simulink model "robotarm_generalization_error"  (R2018b)
settings: Solver=FixedStepAuto  StartTime=0.0  StopTime=10  FixedStep=options.dt  RelTol=1e-3  AbsTol=1e-6
PreLoadFcn:
  | const_ref=-0.1;
  | options.dt=0.02;
libraries: neural x528, simulink x1
(part 6 of 20)

== system robotarm_generalization_error/pre_0/Layer 3/Delays 1 ==
  "p{3}" : Inport  PortDimensions=30
      mask Display: e = 0.06;c1 = [120 230 180]/255;c2 = ([120 230 180]+0)/(256+128);c3 = ([120 230 180]+128)/(256+128);patch([0 1 1 0],[0 0 1 1],c1);patch([0 1 1 1-e 1-e 0+e],[0 0 1 1-e 0+e 0+e],c2);patch([0 0 1 1-e 0+e 0+e],[0 1 1 1-e 1-e 0+e],c3);plot([0 1 1 0 0],[0 0 1 1 0]);
  mux : Mux  Inputs=1
      mask Display: e = 0.06;c1 = [120 150 230]/255;c2 = ([120 150 230]+0)/383;c3 = ([120 150 230]+128)/383;patch([0 1 1 0],[0 0 1 1],c1);patch([0 1 1 1-e 1-e 0+e],[0 0 1 1-e 0+e 0+e],c2);patch([0 0 1 1-e 0+e 0+e],[0 1 1 1-e 1-e 0+e],c3);plot([0 1 1 0 0],[0 0 1 1 0]);disp('Mux')
  "pd{3,2}" : Outport
      mask Display: e = 0.06;c1 = [120 230 180]/255;c2 = ([120 230 180]+0)/(256+128);c3 = ([120 230 180]+128)/(256+128);patch([0 1 1 0],[0 0 1 1],c1);patch([0 1 1 1-e 1-e 0+e],[0 0 1 1-e 0+e 0+e],c2);patch([0 0 1 1-e 0+e 0+e],[0 1 1 1-e 1-e 0+e],c3);plot([0 1 1 0 0],[0 0 1 1 0]);
  wires:
  "p{3}"/1 -> mux/1
  mux/1 -> "pd{3,2}"/1

== system robotarm_generalization_error/pre_0/Layer 3/LW{3,2} ==
  "ad{3,2}" : Inport  PortDimensions=30
      mask Display: e = 0.06;c1 = [120 230 180]/255;c2 = ([120 230 180]+0)/(256+128);c3 = ([120 230 180]+128)/(256+128);patch([0 1 1 0],[0 0 1 1],c1);patch([0 1 1 1-e 1-e 0+e],[0 0 1 1-e 0+e 0+e],c2);patch([0 0 1 1-e 0+e 0+e],[0 1 1 1-e 1-e 0+e],c3);plot([0 1 1 0 0],[0 0 1 1 0]);
  "IW{3,2}(1,:)'" : Constant  Value=[0.1482283738558132502038944267042097635567188262939453125;-0.292502547224109787915580227490863762795925140380859375;-0.50468612294941428420003148858086206018924713134765625;-0.04670559747562709473900355305886478163301944732666015625;-0.041057504134613953539201247622258961200714111328125;-0.047944240213243671799858702797791920602321624755859375;-0.058496921474289344244912314252360374666750431060791015625;0.6148107235436384154780853350530378520488739013671875;0.426521583356435696199326912392280064523220062255859375;-0.07561076580819027503910234599970863200724124908447265625;-0.11443132652669028848091414829468703828752040863037109375;0.0323020095753548119876796818061848171055316925048828125;-0.09697924204691467375827329533422016538679599761962890625;-0.0005858338048831922273418371105435653589665889739990234375;0.401630644371972878037269083506544120609760284423828125;-0.01411896694504084781573993723213789053261280059814453125;0.128668160799946307282226598545094020664691925048828125;0.315585885323380666012127448993851430714130401611328125;0.03498763759822243191166535325464792549610137939453125;0.263939485164793652405279544836957938969135284423828125;-0.04660773546215137008719153755009756423532962799072265625;0.098416358531250913710408667611773125827312469482421875;-0.05026154890612459513743459638135391287505626678466796875;0.5797294681370976920931070708320476114749908447265625;-0.1274272878263316977065500168464495800435543060302734375;0.29329703665639728082936699138372205197811126708984375;-0.20780235218750531256404201485565863549709320068359375;0.1349574147376667310194164883796474896371364593505859375;0.158832086422066420805521147485706023871898651123046875;-0.38523169250914823802389719276106916368007659912109375]
      mask Display: e = 0.06;c1 = [120 150 230]/255;c2 = ([120 150 230]+0)/383;c3 = ([120 150 230]+128)/383;patch([0 1 1 0],[0 0 1 1],c1);patch([0 1 1 1-e 1-e 0+e],[0 0 1 1-e 0+e 0+e],c2);patch([0 0 1 1-e 0+e 0+e],[0 1 1 1-e 1-e 0+e],c3);plot([0 1 1 0 0],[0 0 1 1 0]);disp('weights');
  Mux : Mux  Inputs=1
      mask Display: e = 0.06;c1 = [120 150 230]/255;c2 = ([120 150 230]+0)/383;c3 = ([120 150 230]+128)/383;patch([0 1 1 0],[0 0 1 1],c1);patch([0 1 1 1-e 1-e 0+e],[0 0 1 1-e 0+e 0+e],c2);patch([0 0 1 1-e 0+e 0+e],[0 1 1 1-e 1-e 0+e],c3);plot([0 1 1 0 0],[0 0 1 1 0]);disp('Mux');
  dotprod1 : neural/Weight Functions/dotprod
  "lz{3,2}" : Outport
      mask Display: e = 0.06;c1 = [120 230 180]/255;c2 = ([120 230 180]+0)/(256+128);c3 = ([120 230 180]+128)/(256+128);patch([0 1 1 0],[0 0 1 1],c1);patch([0 1 1 1-e 1-e 0+e],[0 0 1 1-e 0+e 0+e],c2);patch([0 0 1 1-e 0+e 0+e],[0 1 1 1-e 1-e 0+e],c3);plot([0 1 1 0 0],[0 0 1 1 0]);
  wires:
  "IW{3,2}(1,:)'"/1 -> dotprod1/1
  "ad{3,2}"/1 -> dotprod1/2
  dotprod1/1 -> Mux/1
  Mux/1 -> "lz{3,2}"/1

== system robotarm_generalization_error/pre_0.00001/Layer 1/Delays 1 ==
  "p{1}" : Inport  PortDimensions=10
      mask Display: e = 0.06;c1 = [120 230 180]/255;c2 = ([120 230 180]+0)/(256+128);c3 = ([120 230 180]+128)/(256+128);patch([0 1 1 0],[0 0 1 1],c1);patch([0 1 1 1-e 1-e 0+e],[0 0 1 1-e 0+e 0+e],c2);patch([0 0 1 1-e 0+e 0+e],[0 1 1 1-e 1-e 0+e],c3);plot([0 1 1 0 0],[0 0 1 1 0]);
  mux : Mux  Inputs=1
      mask Display: e = 0.06;c1 = [120 150 230]/255;c2 = ([120 150 230]+0)/383;c3 = ([120 150 230]+128)/383;patch([0 1 1 0],[0 0 1 1],c1);patch([0 1 1 1-e 1-e 0+e],[0 0 1 1-e 0+e 0+e],c2);patch([0 0 1 1-e 0+e 0+e],[0 1 1 1-e 1-e 0+e],c3);plot([0 1 1 0 0],[0 0 1 1 0]);disp('Mux')
  "pd{1,1}" : Outport
      mask Display: e = 0.06;c1 = [120 230 180]/255;c2 = ([120 230 180]+0)/(256+128);c3 = ([120 230 180]+128)/(256+128);patch([0 1 1 0],[0 0 1 1],c1);patch([0 1 1 1-e 1-e 0+e],[0 0 1 1-e 0+e 0+e],c2);patch([0 0 1 1-e 0+e 0+e],[0 1 1 1-e 1-e 0+e],c3);plot([0 1 1 0 0],[0 0 1 1 0]);
  wires:
  "p{1}"/1 -> mux/1
  mux/1 -> "pd{1,1}"/1

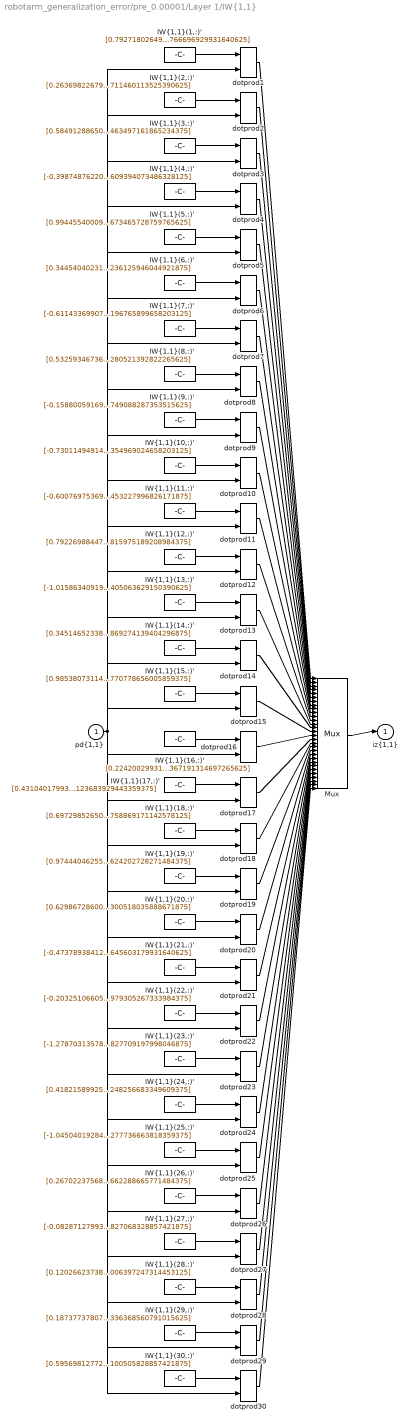
== system robotarm_generalization_error/pre_0.00001/Layer 1/IW{1,1} ==
  "pd{1,1}" : Inport  PortDimensions=10
      mask Display: e = 0.06;c1 = [120 230 180]/255;c2 = ([120 230 180]+0)/(256+128);c3 = ([120 230 180]+128)/(256+128);patch([0 1 1 0],[0 0 1 1],c1);patch([0 1 1 1-e 1-e 0+e],[0 0 1 1-e 0+e 0+e],c2);patch([0 0 1 1-e 0+e 0+e],[0 1 1 1-e 1-e 0+e],c3);plot([0 1 1 0 0],[0 0 1 1 0]);
  "IW{1,1}(1,:)'" : Constant  Value=[0.792718026499978467569462736719287931919097900390625;-0.70093126819101170266179678947082720696926116943359375;0.05608783841132684855335099882722715847194194793701171875;0.650494068864035934751655076979659497737884521484375;0.339334487435024423351848099628114141523838043212890625;0.0859367098609566948397286978433839976787567138671875;-0.00303800444739509879765737565548988641239702701568603515625;0.403054897202263173738856494310311973094940185546875;-0.9987802927080036141660457360558211803436279296875;0.88997533042789600532529448173590935766696929931640625]
      mask Display: e = 0.06;c1 = [120 150 230]/255;c2 = ([120 150 230]+0)/383;c3 = ([120 150 230]+128)/383;patch([0 1 1 0],[0 0 1 1],c1);patch([0 1 1 1-e 1-e 0+e],[0 0 1 1-e 0+e 0+e],c2);patch([0 0 1 1-e 0+e 0+e],[0 1 1 1-e 1-e 0+e],c3);plot([0 1 1 0 0],[0 0 1 1 0]);disp('Weights');
  "IW{1,1}(10,:)'" : Constant  Value=[-0.73011494914437558012565432363771833479404449462890625;0.53826111472537074842392712525906972587108612060546875;-0.91095835698161409244022479470004327595233917236328125;-0.36941848168567614774104868047288618981838226318359375;0.448631007647780022384864651030511595308780670166015625;1.0297337541511095704294120878330431878566741943359375;-0.918213824035238435072869833675213158130645751953125;0.0016459707979491135405869517427390746888704597949981689453125;0.03098860177049818365180300361316767521202564239501953125;0.078742092618516335011946694066864438354969024658203125]
      mask Display: e = 0.06;c1 = [120 150 230]/255;c2 = ([120 150 230]+0)/383;c3 = ([120 150 230]+128)/383;patch([0 1 1 0],[0 0 1 1],c1);patch([0 1 1 1-e 1-e 0+e],[0 0 1 1-e 0+e 0+e],c2);patch([0 0 1 1-e 0+e 0+e],[0 1 1 1-e 1-e 0+e],c3);plot([0 1 1 0 0],[0 0 1 1 0]);disp('Weights');
  "IW{1,1}(11,:)'" : Constant  Value=[-0.60076975369661955728162183731910772621631622314453125;-0.7815534313177094905000785729498602449893951416015625;-0.10636660936180315772947579944229801185429096221923828125;-0.5105893863131518717324297540471889078617095947265625;-0.143121669664646067321456257559475488960742950439453125;0.60572962861191059769083722130744718015193939208984375;-1.0447411499515466548615449937642551958560943603515625;-0.4967530929653134474932585362694226205348968505859375;0.6436329915056864248157353358692489564418792724609375;-0.493380264809257951252874363490263931453227996826171875]
      mask Display: e = 0.06;c1 = [120 150 230]/255;c2 = ([120 150 230]+0)/383;c3 = ([120 150 230]+128)/383;patch([0 1 1 0],[0 0 1 1],c1);patch([0 1 1 1-e 1-e 0+e],[0 0 1 1-e 0+e 0+e],c2);patch([0 0 1 1-e 0+e 0+e],[0 1 1 1-e 1-e 0+e],c3);plot([0 1 1 0 0],[0 0 1 1 0]);disp('Weights');
  "IW{1,1}(12,:)'" : Constant  Value=[0.79226988447897206402359415733371861279010772705078125;0.64150368497529985933880425363895483314990997314453125;0.4266831198942007130625597710604779422283172607421875;0.66813282241212046397293988775345496833324432373046875;0.75696621485603021728394423917052336037158966064453125;1.0631786645748324549032304275897331535816192626953125;0.025638359869932292323113642851240001618862152099609375;-0.401362514161049066530040363431908190250396728515625;-0.95818784785836885742327240222948603332042694091796875;0.70967759913524675052798329488723538815975189208984375]
      mask Display: e = 0.06;c1 = [120 150 230]/255;c2 = ([120 150 230]+0)/383;c3 = ([120 150 230]+128)/383;patch([0 1 1 0],[0 0 1 1],c1);patch([0 1 1 1-e 1-e 0+e],[0 0 1 1-e 0+e 0+e],c2);patch([0 0 1 1-e 0+e 0+e],[0 1 1 1-e 1-e 0+e],c3);plot([0 1 1 0 0],[0 0 1 1 0]);disp('Weights');
  "IW{1,1}(13,:)'" : Constant  Value=[-1.0158634091929668041842660386464558541774749755859375;0.69775822024707412349897595049696974456310272216796875;0.03991779606440941374767561455882969312369823455810546875;0.875077748235802754805945369298569858074188232421875;0.375559951228444599546918425403418950736522674560546875;0.329837496371995164690105184490676037967205047607421875;0.1780538341284050585233700303433579392731189727783203125;-1.1006097630269240372768990710028447210788726806640625;-0.9454926553955613766078158732852898538112640380859375;-0.62445206361746097289966428434127010405063629150390625]
      mask Display: e = 0.06;c1 = [120 150 230]/255;c2 = ([120 150 230]+0)/383;c3 = ([120 150 230]+128)/383;patch([0 1 1 0],[0 0 1 1],c1);patch([0 1 1 1-e 1-e 0+e],[0 0 1 1-e 0+e 0+e],c2);patch([0 0 1 1-e 0+e 0+e],[0 1 1 1-e 1-e 0+e],c3);plot([0 1 1 0 0],[0 0 1 1 0]);disp('Weights');
  "IW{1,1}(14,:)'" : Constant  Value=[0.34514652338435525269488834965159185230731964111328125;-0.2893002995822107070722495336667634546756744384765625;0.373129036692417870302307392194052226841449737548828125;0.43645209584388922063880045243422500789165496826171875;0.5361512855752612605186868677265010774135589599609375;-0.78016467077285167608380334058892913162708282470703125;0.06624618858070906168844516059834859333932399749755859375;0.769506169236554793400273410952650010585784912109375;0.5983570099323409774427773299976252019405364990234375;1.12424455414036827960444497875869274139404296875]
      mask Display: e = 0.06;c1 = [120 150 230]/255;c2 = ([120 150 230]+0)/383;c3 = ([120 150 230]+128)/383;patch([0 1 1 0],[0 0 1 1],c1);patch([0 1 1 1-e 1-e 0+e],[0 0 1 1-e 0+e 0+e],c2);patch([0 0 1 1-e 0+e 0+e],[0 1 1 1-e 1-e 0+e],c3);plot([0 1 1 0 0],[0 0 1 1 0]);disp('Weights');
  "IW{1,1}(15,:)'" : Constant  Value=[0.98538073114240554151166406882111914455890655517578125;-0.2081376007440757514022067198311560787260532379150390625;0.705773248635602090672591657494194805622100830078125;-0.55424090413714910408060632107662968337535858154296875;-0.366114997134839803560879545329953543841838836669921875;0.16451585470810403677432987024076282978057861328125;0.2042206532680158337367259946404374204576015472412109375;0.361942870153160567436856354106566868722438812255859375;0.81392198960292361231694258094648830592632293701171875;-0.04351142751805280040056089774225256405770778656005859375]
      mask Display: e = 0.06;c1 = [120 150 230]/255;c2 = ([120 150 230]+0)/383;c3 = ([120 150 230]+128)/383;patch([0 1 1 0],[0 0 1 1],c1);patch([0 1 1 1-e 1-e 0+e],[0 0 1 1-e 0+e 0+e],c2);patch([0 0 1 1-e 0+e 0+e],[0 1 1 1-e 1-e 0+e],c3);plot([0 1 1 0 0],[0 0 1 1 0]);disp('Weights');
  "IW{1,1}(16,:)'" : Constant  Value=[0.2242002993113756115217682918228092603385448455810546875;0.8059584455887829346210082803736440837383270263671875;0.041800229802249212751608098415090353228151798248291015625;0.60414663903486454099578395471326075494289398193359375;0.472397615412359639375239339642575941979885101318359375;0.734346162971953209108733062748797237873077392578125;-0.752981881277486220227501689805649220943450927734375;0.62057947307669880654401595165836624801158905029296875;0.096505326649476141920303007282200269401073455810546875;0.8622956852991967569010967054055072367191314697265625]
      mask Display: e = 0.06;c1 = [120 150 230]/255;c2 = ([120 150 230]+0)/383;c3 = ([120 150 230]+128)/383;patch([0 1 1 0],[0 0 1 1],c1);patch([0 1 1 1-e 1-e 0+e],[0 0 1 1-e 0+e 0+e],c2);patch([0 0 1 1-e 0+e 0+e],[0 1 1 1-e 1-e 0+e],c3);plot([0 1 1 0 0],[0 0 1 1 0]);disp('Weights');
  "IW{1,1}(17,:)'" : Constant  Value=[0.43104017993212939696690000346279703080654144287109375;-1.0114211457865944776557398654404096305370330810546875;0.529087704281758330893126185401342809200286865234375;0.2176133943608942467040634483055328018963336944580078125;0.1811025579219071313108457843554788269102573394775390625;1.2162624044515830679102919020806439220905303955078125;-0.74319871506040968700546045511146076023578643798828125;-0.1520026511767330335000991681226878426969051361083984375;0.63031088499891152476806155391386710107326507568359375;1.236757817028600214825928560458123683929443359375]
      mask Display: e = 0.06;c1 = [120 150 230]/255;c2 = ([120 150 230]+0)/383;c3 = ([120 150 230]+128)/383;patch([0 1 1 0],[0 0 1 1],c1);patch([0 1 1 1-e 1-e 0+e],[0 0 1 1-e 0+e 0+e],c2);patch([0 0 1 1-e 0+e 0+e],[0 1 1 1-e 1-e 0+e],c3);plot([0 1 1 0 0],[0 0 1 1 0]);disp('Weights');
  "IW{1,1}(18,:)'" : Constant  Value=[0.69729852650166190830560708491248078644275665283203125;0.328669282591977085505874356385902501642704010009765625;-0.7743289263332922001126235045376233756542205810546875;-0.427401450965814333482484244086663238704204559326171875;0.7684882590639843247259932468296028673648834228515625;-0.463323750289418134773455903996364213526248931884765625;0.60292020024025561042435583658516407012939453125;-0.7625519329490850761743558905436657369136810302734375;-1.01656580547610975173711267416365444660186767578125;0.11875693701802410295886858193625812418758869171142578125]
      mask Display: e = 0.06;c1 = [120 150 230]/255;c2 = ([120 150 230]+0)/383;c3 = ([120 150 230]+128)/383;patch([0 1 1 0],[0 0 1 1],c1);patch([0 1 1 1-e 1-e 0+e],[0 0 1 1-e 0+e 0+e],c2);patch([0 0 1 1-e 0+e 0+e],[0 1 1 1-e 1-e 0+e],c3);plot([0 1 1 0 0],[0 0 1 1 0]);disp('Weights');
  "IW{1,1}(19,:)'" : Constant  Value=[0.9744404625544247355861671167076565325260162353515625;-0.443476463011988730755774668068625032901763916015625;0.66053078889701632991915403181337751448154449462890625;0.334011530121419764061130308618885464966297149658203125;-0.65018637595317307908970860808040015399456024169921875;0.1459647843651813714505038888091803528368473052978515625;-0.02049491392940527845212272950448095798492431640625;0.2347202341554484039676253814832307398319244384765625;0.40081420007591461729390402979333885014057159423828125;0.5577229173026141406666056354879401624202728271484375]
      mask Display: e = 0.06;c1 = [120 150 230]/255;c2 = ([120 150 230]+0)/383;c3 = ([120 150 230]+128)/383;patch([0 1 1 0],[0 0 1 1],c1);patch([0 1 1 1-e 1-e 0+e],[0 0 1 1-e 0+e 0+e],c2);patch([0 0 1 1-e 0+e 0+e],[0 1 1 1-e 1-e 0+e],c3);plot([0 1 1 0 0],[0 0 1 1 0]);disp('Weights');
  "IW{1,1}(2,:)'" : Constant  Value=[0.2636982267939718127536252723075449466705322265625;-0.8548952516237184884317912292317487299442291259765625;0.486232191268747004908590270133572630584239959716796875;-0.240014422354133005743648254792788065969944000244140625;-0.262996500397268795357064163908944465219974517822265625;0.130598753997902605750169868770171888172626495361328125;-1.24364530908259585118003087700344622135162353515625;1.042541453544808316422631833120249211788177490234375;-0.266776099155329904366595883402624167501926422119140625;-0.39633402017672347827925705132656730711460113525390625]
      mask Display: e = 0.06;c1 = [120 150 230]/255;c2 = ([120 150 230]+0)/383;c3 = ([120 150 230]+128)/383;patch([0 1 1 0],[0 0 1 1],c1);patch([0 1 1 1-e 1-e 0+e],[0 0 1 1-e 0+e 0+e],c2);patch([0 0 1 1-e 0+e 0+e],[0 1 1 1-e 1-e 0+e],c3);plot([0 1 1 0 0],[0 0 1 1 0]);disp('Weights');
  "IW{1,1}(20,:)'" : Constant  Value=[0.62986728600408403710986249279812909662723541259765625;0.01225817241564213823379336787411375553347170352935791015625;-0.54365738659735018956098429043777287006378173828125;0.7513404595413641917645009016268886625766754150390625;-0.440534965778207443509728591379825957119464874267578125;0.8029930625960999268642126480699516832828521728515625;0.1315056605710212267457137613746454007923603057861328125;0.394492629501052072260591785379801876842975616455078125;-0.9914979463203772436230565290316008031368255615234375;-0.08105902260661372593641971207034657709300518035888671875]
      mask Display: e = 0.06;c1 = [120 150 230]/255;c2 = ([120 150 230]+0)/383;c3 = ([120 150 230]+128)/383;patch([0 1 1 0],[0 0 1 1],c1);patch([0 1 1 1-e 1-e 0+e],[0 0 1 1-e 0+e 0+e],c2);patch([0 0 1 1-e 0+e 0+e],[0 1 1 1-e 1-e 0+e],c3);plot([0 1 1 0 0],[0 0 1 1 0]);disp('Weights');
  "IW{1,1}(21,:)'" : Constant  Value=[-0.47378938412666349311308522374019958078861236572265625;0.48578761228713374098475696882815100252628326416015625;0.034475295389157438463723082122669438831508159637451171875;0.155503246769882752520430813092389144003391265869140625;-0.92743067868098372219520797443692572414875030517578125;0.99469786221565303918623612844385206699371337890625;-0.88054678970821675942914907864178530871868133544921875;0.588651768692387999948323340504430234432220458984375;-0.1923798942803716383043166615607333369553089141845703125;-0.73935992594295785185209979317733086645603179931640625]
      mask Display: e = 0.06;c1 = [120 150 230]/255;c2 = ([120 150 230]+0)/383;c3 = ([120 150 230]+128)/383;patch([0 1 1 0],[0 0 1 1],c1);patch([0 1 1 1-e 1-e 0+e],[0 0 1 1-e 0+e 0+e],c2);patch([0 0 1 1-e 0+e 0+e],[0 1 1 1-e 1-e 0+e],c3);plot([0 1 1 0 0],[0 0 1 1 0]);disp('Weights');
  "IW{1,1}(22,:)'" : Constant  Value=[-0.203251066050530393436446274790796451270580291748046875;0.6801901609191822739575172818149439990520477294921875;0.273506231817061296052173702264553867280483245849609375;0.49567466965405027057300912929349578917026519775390625;-0.5401198371168847156553738386719487607479095458984375;-0.62218739456634530871070865032379515469074249267578125;1.229200213576618683219976446707732975482940673828125;0.1471868028976376086003341470131999813020229339599609375;-0.647144509544419488378252935945056378841400146484375;-0.94927323473495250905074271940975449979305267333984375]
      mask Display: e = 0.06;c1 = [120 150 230]/255;c2 = ([120 150 230]+0)/383;c3 = ([120 150 230]+128)/383;patch([0 1 1 0],[0 0 1 1],c1);patch([0 1 1 1-e 1-e 0+e],[0 0 1 1-e 0+e 0+e],c2);patch([0 0 1 1-e 0+e 0+e],[0 1 1 1-e 1-e 0+e],c3);plot([0 1 1 0 0],[0 0 1 1 0]);disp('Weights');
  "IW{1,1}(23,:)'" : Constant  Value=[-1.278703135784561961685312780900858342647552490234375;-0.3235779278436548000996708651655353605747222900390625;0.95102036510107457178975209899363107979297637939453125;0.5361783260187056310286379812168888747692108154296875;-0.7378988594593567373891573879518546164035797119140625;0.2318410310548441877198655447500641457736492156982421875;-0.00098105012836622739087755196152329517644830048084259033203125;0.11502282741329851456502098017153912223875522613525390625;0.30763215325637982555662119921180419623851776123046875;-0.37808630590338931920513232398661784827709197998046875]
      mask Display: e = 0.06;c1 = [120 150 230]/255;c2 = ([120 150 230]+0)/383;c3 = ([120 150 230]+128)/383;patch([0 1 1 0],[0 0 1 1],c1);patch([0 1 1 1-e 1-e 0+e],[0 0 1 1-e 0+e 0+e],c2);patch([0 0 1 1-e 0+e 0+e],[0 1 1 1-e 1-e 0+e],c3);plot([0 1 1 0 0],[0 0 1 1 0]);disp('Weights');
  "IW{1,1}(24,:)'" : Constant  Value=[0.418215899254464840151257476463797502219676971435546875;-0.67449721806075346730580122311948798596858978271484375;0.52895924674882233151862465092563070356845855712890625;-0.3918847743765019320250075907097198069095611572265625;-1.4710418700029499472492489076103083789348602294921875;0.988510203554212818488622360746376216411590576171875;-0.277304749265782690681447775205015204846858978271484375;0.2465694150963897157691206984964082948863506317138671875;-0.6082144905269319945517736414331011474132537841796875;-0.379177860511200781612473065251833759248256683349609375]
      mask Display: e = 0.06;c1 = [120 150 230]/255;c2 = ([120 150 230]+0)/383;c3 = ([120 150 230]+128)/383;patch([0 1 1 0],[0 0 1 1],c1);patch([0 1 1 1-e 1-e 0+e],[0 0 1 1-e 0+e 0+e],c2);patch([0 0 1 1-e 0+e 0+e],[0 1 1 1-e 1-e 0+e],c3);plot([0 1 1 0 0],[0 0 1 1 0]);disp('Weights');
  "IW{1,1}(25,:)'" : Constant  Value=[-1.0450401928464863043899413241888396441936492919921875;0.26768904396254178390535116704995743930339813232421875;0.6220878362540105399602907709777355194091796875;-0.44542176550071765905869369817082770168781280517578125;-0.42519305307979815555796676562749780714511871337890625;0.5075149011143402777435085226898081600666046142578125;0.341217779421175981813263433650718070566654205322265625;0.7142429533366334570843036999576725065708160400390625;-0.246923154742340000833422664072713814675807952880859375;-0.45704099877693804554468215428641997277736663818359375]
      mask Display: e = 0.06;c1 = [120 150 230]/255;c2 = ([120 150 230]+0)/383;c3 = ([120 150 230]+128)/383;patch([0 1 1 0],[0 0 1 1],c1);patch([0 1 1 1-e 1-e 0+e],[0 0 1 1-e 0+e 0+e],c2);patch([0 0 1 1-e 0+e 0+e],[0 1 1 1-e 1-e 0+e],c3);plot([0 1 1 0 0],[0 0 1 1 0]);disp('Weights');
  "IW{1,1}(26,:)'" : Constant  Value=[0.26702237568866371564269002192304469645023345947265625;-0.69680980665157410403054427661118097603321075439453125;-0.882749403982257430101299178204499185085296630859375;0.65580656856601537985085315085598267614841461181640625;-0.77663248582784671913969987144810147583484649658203125;-0.52846124031789531994007802495616488158702850341796875;0.4728223633643595658071490106522105634212493896484375;-0.284166508346968826881351333213387988507747650146484375;-0.365092388405338308388081713928841054439544677734375;-0.26294778754011660648615134050487540662288665771484375]
      mask Display: e = 0.06;c1 = [120 150 230]/255;c2 = ([120 150 230]+0)/383;c3 = ([120 150 230]+128)/383;patch([0 1 1 0],[0 0 1 1],c1);patch([0 1 1 1-e 1-e 0+e],[0 0 1 1-e 0+e 0+e],c2);patch([0 0 1 1-e 0+e 0+e],[0 1 1 1-e 1-e 0+e],c3);plot([0 1 1 0 0],[0 0 1 1 0]);disp('Weights');
  "IW{1,1}(27,:)'" : Constant  Value=[-0.08287127993780074586283035387168638408184051513671875;0.7875430051250147389652056517661549150943756103515625;0.0168491671371741348617323552616653614677488803863525390625;-0.58340432971275235640717937712906859815120697021484375;0.34377938651103701062083928263746201992034912109375;-0.94533239146287895149356472757062874734401702880859375;-0.87678431634149822659907158595160581171512603759765625;-0.03627916796862896975373047325774678029119968414306640625;-0.417358344921300528085339465178549289703369140625;0.043483777940783889526255023838530178181827068328857421875]
      mask Display: e = 0.06;c1 = [120 150 230]/255;c2 = ([120 150 230]+0)/383;c3 = ([120 150 230]+128)/383;patch([0 1 1 0],[0 0 1 1],c1);patch([0 1 1 1-e 1-e 0+e],[0 0 1 1-e 0+e 0+e],c2);patch([0 0 1 1-e 0+e 0+e],[0 1 1 1-e 1-e 0+e],c3);plot([0 1 1 0 0],[0 0 1 1 0]);disp('Weights');
  "IW{1,1}(28,:)'" : Constant  Value=[0.12026623738084031567385778771495097316801548004150390625;-0.08928644028343395155911110805391217581927776336669921875;-0.05648596192922143710557492113366606645286083221435546875;-0.1646184924019922224402989741065539419651031494140625;-0.92959219471081755425956316685187630355358123779296875;1.295556872011456750470870247227139770984649658203125;-0.414342322430311604808395031795953400433063507080078125;-0.7872200705337280002282795976498164236545562744140625;0.5688710172331756798058677304652519524097442626953125;-0.172808643670952666315798751384136267006397247314453125]
      mask Display: e = 0.06;c1 = [120 150 230]/255;c2 = ([120 150 230]+0)/383;c3 = ([120 150 230]+128)/383;patch([0 1 1 0],[0 0 1 1],c1);patch([0 1 1 1-e 1-e 0+e],[0 0 1 1-e 0+e 0+e],c2);patch([0 0 1 1-e 0+e 0+e],[0 1 1 1-e 1-e 0+e],c3);plot([0 1 1 0 0],[0 0 1 1 0]);disp('Weights');
  "IW{1,1}(29,:)'" : Constant  Value=[0.1873773780717154779917876794570474885404109954833984375;-0.89952207513065418620357149848132394254207611083984375;0.02928054761829000651740528837763122282922267913818359375;0.43376052047927127208737374530755914747714996337890625;-0.06688360718705747831602792530247825197875499725341796875;0.30697863938615699286316385041573084890842437744140625;-0.398505407718623916313305244329967536032199859619140625;0.0027768963076735355723079212708626073435880243778228759765625;-0.90920184212434218551379672135226428508758544921875;0.81823230580651884480403168709017336368560791015625]
      mask Display: e = 0.06;c1 = [120 150 230]/255;c2 = ([120 150 230]+0)/383;c3 = ([120 150 230]+128)/383;patch([0 1 1 0],[0 0 1 1],c1);patch([0 1 1 1-e 1-e 0+e],[0 0 1 1-e 0+e 0+e],c2);patch([0 0 1 1-e 0+e 0+e],[0 1 1 1-e 1-e 0+e],c3);plot([0 1 1 0 0],[0 0 1 1 0]);disp('Weights');
  "IW{1,1}(3,:)'" : Constant  Value=[0.584912886502609641325989286997355520725250244140625;0.037499839273540190587308273961753002367913722991943359375;0.1559421387207623188597693797419196926057338714599609375;-0.40430179886704864511415280503570102155208587646484375;-0.73667631815217238244741793096181936562061309814453125;0.88611514021734993917789324768818914890289306640625;0.7688638706773576192432528841891326010227203369140625;-0.458789132619995931872125538575346581637859344482421875;0.05033716620315238643446065225361962802708148956298828125;0.519669574114098420380969400866888463497161865234375]
      mask Display: e = 0.06;c1 = [120 150 230]/255;c2 = ([120 150 230]+0)/383;c3 = ([120 150 230]+128)/383;patch([0 1 1 0],[0 0 1 1],c1);patch([0 1 1 1-e 1-e 0+e],[0 0 1 1-e 0+e 0+e],c2);patch([0 0 1 1-e 0+e 0+e],[0 1 1 1-e 1-e 0+e],c3);plot([0 1 1 0 0],[0 0 1 1 0]);disp('Weights');
  "IW{1,1}(30,:)'" : Constant  Value=[0.5956981277261983453996663229190744459629058837890625;0.257980583125774265429441811647848226130008697509765625;-0.093553679947365353530841503015835769474506378173828125;0.681955696995973692509096508729271590709686279296875;-0.404027881545070244317940932887722738087177276611328125;-0.76807032630568994324704590326291508972644805908203125;1.0526870101417660219311756009119562804698944091796875;0.80168802925118309854468634512159042060375213623046875;0.36198320668787331566562670559505932033061981201171875;0.7228496620328506150343628178234212100505828857421875]
      mask Display: e = 0.06;c1 = [120 150 230]/255;c2 = ([120 150 230]+0)/383;c3 = ([120 150 230]+128)/383;patch([0 1 1 0],[0 0 1 1],c1);patch([0 1 1 1-e 1-e 0+e],[0 0 1 1-e 0+e 0+e],c2);patch([0 0 1 1-e 0+e 0+e],[0 1 1 1-e 1-e 0+e],c3);plot([0 1 1 0 0],[0 0 1 1 0]);disp('Weights');
  "IW{1,1}(4,:)'" : Constant  Value=[-0.3987487622019754152091763899079523980617523193359375;0.3639334878667723760514718378544785082340240478515625;0.55073689900528954854763696857844479382038116455078125;-0.70170443549172600850027947672060690820217132568359375;-0.69772627901864769928153009459492750465869903564453125;0.0801987147770017172465628618738264776766300201416015625;0.1123547017193594343975604488150565885007381439208984375;-0.89958941764986477540588793999631889164447784423828125;-0.51186634104249784105178378013079054653644561767578125;0.395166862904763604991131842325557954609394073486328125]
      mask Display: e = 0.06;c1 = [120 150 230]/255;c2 = ([120 150 230]+0)/383;c3 = ([120 150 230]+128)/383;patch([0 1 1 0],[0 0 1 1],c1);patch([0 1 1 1-e 1-e 0+e],[0 0 1 1-e 0+e 0+e],c2);patch([0 0 1 1-e 0+e 0+e],[0 1 1 1-e 1-e 0+e],c3);plot([0 1 1 0 0],[0 0 1 1 0]);disp('Weights');
  "IW{1,1}(5,:)'" : Constant  Value=[0.9944554000969259011100120915216393768787384033203125;0.43366553125329254658737454519723542034626007080078125;0.2435987442017230886204259832084062509238719940185546875;-0.57916599317854655648574180304422043263912200927734375;-0.76993312696056948052358848144649527966976165771484375;1.337585755268572373921642792993225157260894775390625;-0.10896606782235758459354002525287796743214130401611328125;0.38956849666204440563177513467962853610515594482421875;-0.61855439925363298048210936030955053865909576416015625;-0.289724171169875310827279690784052945673465728759765625]
      mask Display: e = 0.06;c1 = [120 150 230]/255;c2 = ([120 150 230]+0)/383;c3 = ([120 150 230]+128)/383;patch([0 1 1 0],[0 0 1 1],c1);patch([0 1 1 1-e 1-e 0+e],[0 0 1 1-e 0+e 0+e],c2);patch([0 0 1 1-e 0+e 0+e],[0 1 1 1-e 1-e 0+e],c3);plot([0 1 1 0 0],[0 0 1 1 0]);disp('Weights');
  "IW{1,1}(6,:)'" : Constant  Value=[0.344540402319315874901661800322472117841243743896484375;0.8087571993076443366277317181811667978763580322265625;0.1975205012380635560820252294433885253965854644775390625;0.7169620962620346649174507547286339104175567626953125;-0.43602709995182820090775521748582832515239715576171875;-0.1796510465245913235055041923260432668030261993408203125;-0.1442507592862380672027455830175313167273998260498046875;-0.1427612994063457707571984656169661320745944976806640625;-0.54819875015861974087982844139332883059978485107421875;-0.190915684066005564289980611647479236125946044921875]
      mask Display: e = 0.06;c1 = [120 150 230]/255;c2 = ([120 150 230]+0)/383;c3 = ([120 150 230]+128)/383;patch([0 1 1 0],[0 0 1 1],c1);patch([0 1 1 1-e 1-e 0+e],[0 0 1 1-e 0+e 0+e],c2);patch([0 0 1 1-e 0+e 0+e],[0 1 1 1-e 1-e 0+e],c3);plot([0 1 1 0 0],[0 0 1 1 0]);disp('Weights');
  "IW{1,1}(7,:)'" : Constant  Value=[-0.61143369907137123941964773621293716132640838623046875;-0.14240540271073809375224072937271557748317718505859375;-0.54474721016627769554219185010879300534725189208984375;-0.5765566045200163358686040737666189670562744140625;-1.3944510232538387395351264785858802497386932373046875;0.972976043687458602704509758041240274906158447265625;-0.373034909650978352413375205287593416869640350341796875;0.16736266310817249358677827331121079623699188232421875;0.5714355452905375276628774372511543333530426025390625;-0.417661462847210895876770564427715726196765899658203125]
      mask Display: e = 0.06;c1 = [120 150 230]/255;c2 = ([120 150 230]+0)/383;c3 = ([120 150 230]+128)/383;patch([0 1 1 0],[0 0 1 1],c1);patch([0 1 1 1-e 1-e 0+e],[0 0 1 1-e 0+e 0+e],c2);patch([0 0 1 1-e 0+e 0+e],[0 1 1 1-e 1-e 0+e],c3);plot([0 1 1 0 0],[0 0 1 1 0]);disp('Weights');
  "IW{1,1}(8,:)'" : Constant  Value=[0.53259346736689128221087230485863983631134033203125;-0.76988156180607825174178060478880070149898529052734375;0.81533715384688598692974892401252873241901397705078125;0.41358838598987179846488970724749378859996795654296875;0.565382799537205382733873193501494824886322021484375;-0.59193382506844915980082078021951019763946533203125;0.74192295556009579815537335889530368149280548095703125;-0.53108951843921559099470641740481369197368621826171875;-0.448115717205940400358343822517781518399715423583984375;0.1324299116223477401632635519490577280521392822265625]
      mask Display: e = 0.06;c1 = [120 150 230]/255;c2 = ([120 150 230]+0)/383;c3 = ([120 150 230]+128)/383;patch([0 1 1 0],[0 0 1 1],c1);patch([0 1 1 1-e 1-e 0+e],[0 0 1 1-e 0+e 0+e],c2);patch([0 0 1 1-e 0+e 0+e],[0 1 1 1-e 1-e 0+e],c3);plot([0 1 1 0 0],[0 0 1 1 0]);disp('Weights');
  "IW{1,1}(9,:)'" : Constant  Value=[-0.158800591690646364373407095627044327557086944580078125;-0.9799390453563063818620548772742040455341339111328125;0.38909042705299390352280397564754821360111236572265625;0.07975402186501490131576019848580472171306610107421875;0.54029892868337248135190975517616607248783111572265625;1.3739320300820978548728135137935169041156768798828125;-0.281829778295719368674809857111540623009204864501953125;0.01132213122425405893434202653224929235875606536865234375;0.5428933424292214926509814176824875175952911376953125;0.0556212861801359537139433086849749088287353515625]
      mask Display: e = 0.06;c1 = [120 150 230]/255;c2 = ([120 150 230]+0)/383;c3 = ([120 150 230]+128)/383;patch([0 1 1 0],[0 0 1 1],c1);patch([0 1 1 1-e 1-e 0+e],[0 0 1 1-e 0+e 0+e],c2);patch([0 0 1 1-e 0+e 0+e],[0 1 1 1-e 1-e 0+e],c3);plot([0 1 1 0 0],[0 0 1 1 0]);disp('Weights');
  Mux : Mux  Inputs=30
      mask Display: e = 0.06;c1 = [120 150 230]/255;c2 = ([120 150 230]+0)/383;c3 = ([120 150 230]+128)/383;patch([0 1 1 0],[0 0 1 1],c1);patch([0 1 1 1-e 1-e 0+e],[0 0 1 1-e 0+e 0+e],c2);patch([0 0 1 1-e 0+e 0+e],[0 1 1 1-e 1-e 0+e],c3);plot([0 1 1 0 0],[0 0 1 1 0]);disp('Mux');
  dotprod{1..30} (30 alike) : neural/Weight Functions/dotprod
  "iz{1,1}" : Outport
      mask Display: e = 0.06;c1 = [120 230 180]/255;c2 = ([120 230 180]+0)/(256+128);c3 = ([120 230 180]+128)/(256+128);patch([0 1 1 0],[0 0 1 1],c1);patch([0 1 1 1-e 1-e 0+e],[0 0 1 1-e 0+e 0+e],c2);patch([0 0 1 1-e 0+e 0+e],[0 1 1 1-e 1-e 0+e],c3);plot([0 1 1 0 0],[0 0 1 1 0]);
  wires:
  "IW{1,1}(1,:)'"/1 -> dotprod1/1
  "pd{1,1}"/1 -> dotprod1/2, dotprod2/2, dotprod3/2, dotprod4/2, dotprod5/2, dotprod6/2, dotprod7/2, dotprod8/2, dotprod9/2, dotprod10/2, dotprod11/2, dotprod12/2, dotprod13/2, dotprod14/2, dotprod15/2, dotprod16/2, dotprod17/2, dotprod18/2, dotprod19/2, dotprod20/2, dotprod21/2, dotprod22/2, dotprod23/2, dotprod24/2, dotprod25/2, dotprod26/2, dotprod27/2, dotprod28/2, dotprod29/2, dotprod30/2
  dotprod1/1 -> Mux/1
  "IW{1,1}(2,:)'"/1 -> dotprod2/1
  dotprod2/1 -> Mux/2
  "IW{1,1}(3,:)'"/1 -> dotprod3/1
  dotprod3/1 -> Mux/3
  "IW{1,1}(4,:)'"/1 -> dotprod4/1
  dotprod4/1 -> Mux/4
  "IW{1,1}(5,:)'"/1 -> dotprod5/1
  dotprod5/1 -> Mux/5
  "IW{1,1}(6,:)'"/1 -> dotprod6/1
  dotprod6/1 -> Mux/6
  "IW{1,1}(7,:)'"/1 -> dotprod7/1
  dotprod7/1 -> Mux/7
  "IW{1,1}(8,:)'"/1 -> dotprod8/1
  dotprod8/1 -> Mux/8
  "IW{1,1}(9,:)'"/1 -> dotprod9/1
  dotprod9/1 -> Mux/9
  "IW{1,1}(10,:)'"/1 -> dotprod10/1
  dotprod10/1 -> Mux/10
  "IW{1,1}(11,:)'"/1 -> dotprod11/1
  dotprod11/1 -> Mux/11
  "IW{1,1}(12,:)'"/1 -> dotprod12/1
  dotprod12/1 -> Mux/12
  "IW{1,1}(13,:)'"/1 -> dotprod13/1
  dotprod13/1 -> Mux/13
  "IW{1,1}(14,:)'"/1 -> dotprod14/1
  dotprod14/1 -> Mux/14
  "IW{1,1}(15,:)'"/1 -> dotprod15/1
  dotprod15/1 -> Mux/15
  "IW{1,1}(16,:)'"/1 -> dotprod16/1
  dotprod16/1 -> Mux/16
  "IW{1,1}(17,:)'"/1 -> dotprod17/1
  dotprod17/1 -> Mux/17
  "IW{1,1}(18,:)'"/1 -> dotprod18/1
  dotprod18/1 -> Mux/18
  "IW{1,1}(19,:)'"/1 -> dotprod19/1
  dotprod19/1 -> Mux/19
  "IW{1,1}(20,:)'"/1 -> dotprod20/1
  dotprod20/1 -> Mux/20
  "IW{1,1}(21,:)'"/1 -> dotprod21/1
  dotprod21/1 -> Mux/21
  "IW{1,1}(22,:)'"/1 -> dotprod22/1
  dotprod22/1 -> Mux/22
  "IW{1,1}(23,:)'"/1 -> dotprod23/1
  dotprod23/1 -> Mux/23
  "IW{1,1}(24,:)'"/1 -> dotprod24/1
  dotprod24/1 -> Mux/24
  "IW{1,1}(25,:)'"/1 -> dotprod25/1
  dotprod25/1 -> Mux/25
  "IW{1,1}(26,:)'"/1 -> dotprod26/1
  dotprod26/1 -> Mux/26
  "IW{1,1}(27,:)'"/1 -> dotprod27/1
  dotprod27/1 -> Mux/27
  "IW{1,1}(28,:)'"/1 -> dotprod28/1
  dotprod28/1 -> Mux/28
  "IW{1,1}(29,:)'"/1 -> dotprod29/1
  dotprod29/1 -> Mux/29
  "IW{1,1}(30,:)'"/1 -> dotprod30/1
  dotprod30/1 -> Mux/30
  Mux/1 -> "iz{1,1}"/1

== system robotarm_generalization_error/pre_0.00001/Layer 2/Delays 1 ==
  "p{2}" : Inport  PortDimensions=30
      mask Display: e = 0.06;c1 = [120 230 180]/255;c2 = ([120 230 180]+0)/(256+128);c3 = ([120 230 180]+128)/(256+128);patch([0 1 1 0],[0 0 1 1],c1);patch([0 1 1 1-e 1-e 0+e],[0 0 1 1-e 0+e 0+e],c2);patch([0 0 1 1-e 0+e 0+e],[0 1 1 1-e 1-e 0+e],c3);plot([0 1 1 0 0],[0 0 1 1 0]);
  mux : Mux  Inputs=1
      mask Display: e = 0.06;c1 = [120 150 230]/255;c2 = ([120 150 230]+0)/383;c3 = ([120 150 230]+128)/383;patch([0 1 1 0],[0 0 1 1],c1);patch([0 1 1 1-e 1-e 0+e],[0 0 1 1-e 0+e 0+e],c2);patch([0 0 1 1-e 0+e 0+e],[0 1 1 1-e 1-e 0+e],c3);plot([0 1 1 0 0],[0 0 1 1 0]);disp('Mux')
  "pd{2,1}" : Outport
      mask Display: e = 0.06;c1 = [120 230 180]/255;c2 = ([120 230 180]+0)/(256+128);c3 = ([120 230 180]+128)/(256+128);patch([0 1 1 0],[0 0 1 1],c1);patch([0 1 1 1-e 1-e 0+e],[0 0 1 1-e 0+e 0+e],c2);patch([0 0 1 1-e 0+e 0+e],[0 1 1 1-e 1-e 0+e],c3);plot([0 1 1 0 0],[0 0 1 1 0]);
  wires:
  "p{2}"/1 -> mux/1
  mux/1 -> "pd{2,1}"/1
